simulink model "MultiLoop_mode1"  (Simulink 10.1)
settings: Solver=ode45  StartTime=0.0  StopTime=400  FixedStep=Ts_base  MinStep=1e-6  RelTol=1e-6
PreLoadFcn:
  | Mode_1_Init
StopFcn:
  | TEplot
values from neighbouring files (symbols this model uses):
  att_delay = 19.5    [convert_poison.m]
  att_idx = 1    [convert_poison.m]
  att_len = 3.0    (= 3)    [convert_poison.m]
  att_level = 22.9    [convert_poison.m]
  attack_gen_mode = 0    [convert_poison.m]
  n_poisons = 0    [convert_poison.m]
  poison_len = period * 5    (= 35.25)    [convert_poison.m]
  poisons = zeros( np, plen_ticks )    [convert_poison.m]
undefined symbols (not defined in the file or in its folder): r1_0, r4_0, Ts_base, Ts_save
libraries: TElib x17
settings Model: Creator=ricker  LastModifiedBy=mkrav  PacingRate=1.100000
settings DataIOCC: LoadInitialState=on  SaveFinalState=on  SaveFormat=Structure  SignalLoggingSaveFormat=ModelDataLogs  SaveOutput=off  SignalLogging=off  SaveTime=off  SignalLoggingName=sigsOut
settings OptimizationCC: InitFltsAndDblsToZero=on
settings DebuggingCC: SaveWithParameterizedLinksMsg=none  SignalResolutionControl=TryResolveAllWithWarning  MultiTaskDSMMsg=warning  MultiTaskCondExecSysMsg=none  FcnCallInpInsideContextMsg=warning
settings HardwareCC: TargetUnknown=on
settings GRTTargetCC: TargetFcnLib=ansi_tfl_tmw.mat
settings ConfigComp: CovSFcnEnable=off

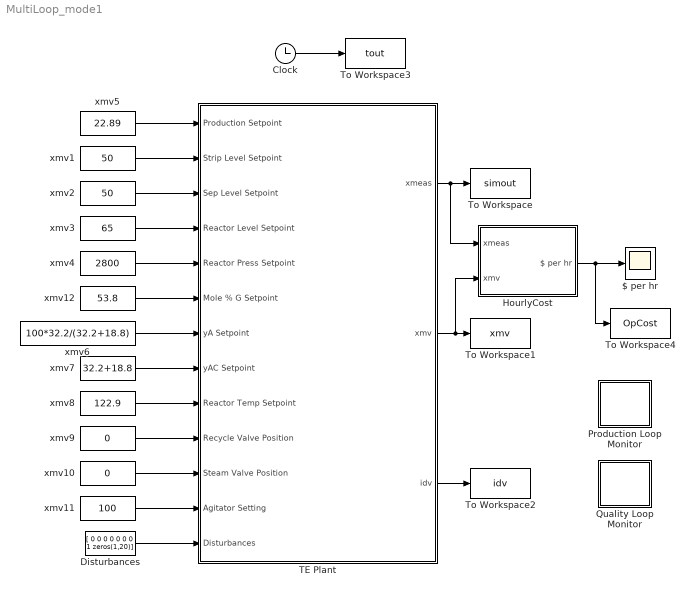
== system MultiLoop_mode1 ==
  $ per hr : Scope
  Clock : Clock
  Disturbances : Constant  Value=[ 0 0 0 0 0 0 0 1 zeros(1,20)]
  HourlyCost : Subsystem
  Production Loop Monitor : Subsystem
  Quality Loop Monitor : Subsystem
  TE Plant : Subsystem
  To Workspace : ToWorkspace  VariableName=simout  SampleTime=Ts_save
  To Workspace1 : ToWorkspace  VariableName=xmv  SampleTime=Ts_save
  To Workspace2 : ToWorkspace  VariableName=idv  SampleTime=Ts_save
  To Workspace3 : ToWorkspace  VariableName=tout  SampleTime=Ts_save
  To Workspace4 : ToWorkspace  VariableName=OpCost  SampleTime=Ts_save
  xmv1 : Constant  Value=50
  xmv10 : Constant  Value=0
  xmv11 : Constant  Value=100
  xmv12 : Constant  Value=53.8
  xmv2 : Constant  Value=50
  xmv3 : Constant  Value=65
  xmv4 : Constant  Value=2800
  xmv5 : Constant  Value=22.89
  xmv6 : Constant  Value=100*32.2/(32.2+18.8)
  xmv7 : Constant  Value=32.2+18.8
  xmv8 : Constant  Value=122.9
  xmv9 : Constant  Value=0
  wires:
  TE Plant/1(xmeas) -> To Workspace/1, HourlyCost/1(xmeas)
  xmv1/1 -> TE Plant/2(Strip Level Setpoint)
  xmv2/1 -> TE Plant/3(Sep Level Setpoint)
  xmv3/1 -> TE Plant/4(Reactor Level Setpoint)
  xmv4/1 -> TE Plant/5(Reactor Press Setpoint)
  xmv8/1 -> TE Plant/9(Reactor Temp Setpoint)
  xmv6/1 -> TE Plant/7(yA Setpoint)
  xmv7/1 -> TE Plant/8(yAC Setpoint)
  TE Plant/2(xmv) -> To Workspace1/1, HourlyCost/2(xmv)
  TE Plant/3(idv) -> To Workspace2/1
  Clock/1 -> To Workspace3/1
  HourlyCost/1($ per hr) -> $ per hr/1, To Workspace4/1
  xmv9/1 -> TE Plant/10(Recycle Valve Position)
  xmv10/1 -> TE Plant/11(Steam Valve Position)
  xmv11/1 -> TE Plant/12(Agitator Setting)
  Disturbances/1 -> TE Plant/13(Disturbances)
  xmv12/1 -> TE Plant/6(Mole % G Setpoint)
  xmv5/1 -> TE Plant/1(Production Setpoint)

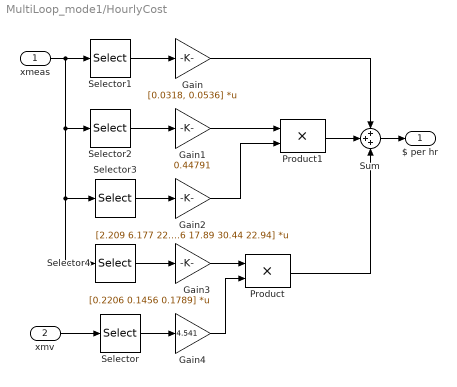
== system MultiLoop_mode1/HourlyCost ==
  xmeas : Inport  PortDimensions=41
  xmv : Inport  Port=2  PortDimensions=12
  Gain : Gain  Gain=[0.0318, 0.0536]  Multiplication=Matrix(K*u)  SaturateOnIntegerOverflow=on  OutDataTypeStr=Inherit: Same as input  ParamDataTypeStr=Inherit: Same as input
  Gain1 : Gain  Gain=0.44791  SaturateOnIntegerOverflow=on  OutDataTypeStr=Inherit: Same as input  ParamDataTypeStr=Inherit: Same as input
  Gain2 : Gain  Gain=[2.209 6.177 22.06 14.56 17.89 30.44 22.94]  Multiplication=Matrix(K*u)  SaturateOnIntegerOverflow=on  OutDataTypeStr=Inherit: Same as input  ParamDataTypeStr=Inherit: Same as input
  Gain3 : Gain  Gain=[0.2206 0.1456 0.1789]  Multiplication=Matrix(K*u)  SaturateOnIntegerOverflow=on  OutDataTypeStr=Inherit: Same as input  ParamDataTypeStr=Inherit: Same as input
  Gain4 : Gain  Gain=4.541  SaturateOnIntegerOverflow=on  OutDataTypeStr=Inherit: Same as input  ParamDataTypeStr=Inherit: Same as input
  Product : Product  SaturateOnIntegerOverflow=on  OutDataTypeStr=Inherit: Same as first input
  Product1 : Product  SaturateOnIntegerOverflow=on  OutDataTypeStr=Inherit: Same as first input
  Selector : Selector  InputPortWidth=12  IndexOptions=Index vector (dialog)  Indices=8  OutputSizes=1
  Selector1 : Selector  InputPortWidth=41  IndexOptions=Index vector (dialog)  Indices=[19 20]  OutputSizes=1
  Selector2 : Selector  InputPortWidth=41  IndexOptions=Index vector (dialog)  Indices=[10]  OutputSizes=1
  Selector3 : Selector  InputPortWidth=41  IndexOptions=Index vector (dialog)  Indices=[29, 31:36]  OutputSizes=1
  Selector4 : Selector  InputPortWidth=41  IndexOptions=Index vector (dialog)  Indices=[37:39]  OutputSizes=1
  Sum : Sum  Inputs=+++  SaturateOnIntegerOverflow=on
  $ per hr : Outport
  wires:
  xmv/1 -> Selector/1
  xmeas/1 -> Selector1/1, Selector2/1, Selector3/1, Selector4/1
  Selector1/1 -> Gain/1
  Selector2/1 -> Gain1/1
  Selector3/1 -> Gain2/1
  Selector4/1 -> Gain3/1
  Selector/1 -> Gain4/1
  Gain3/1 -> Product/1
  Gain4/1 -> Product/2
  Sum/1 -> $ per hr/1
  Product/1 -> Sum/3
  Gain/1 -> Sum/1
  Product1/1 -> Sum/2
  Gain1/1 -> Product1/1
  Gain2/1 -> Product1/2

== system MultiLoop_mode1/Production Loop Monitor ==
  Mux2 : Mux  Inputs=2
  Production : Scope
  wires:
  Mux2/1 -> Production/1
  [xmeas17] -> Mux2/2
  [Prodsp] -> Mux2/1

== system MultiLoop_mode1/Quality Loop Monitor ==
  Mux2 : Mux  Inputs=2
  Quality : Scope
  wires:
  [PctGsp] -> Mux2/1
  [xmeas40] -> Mux2/2
  Mux2/1 -> Quality/1

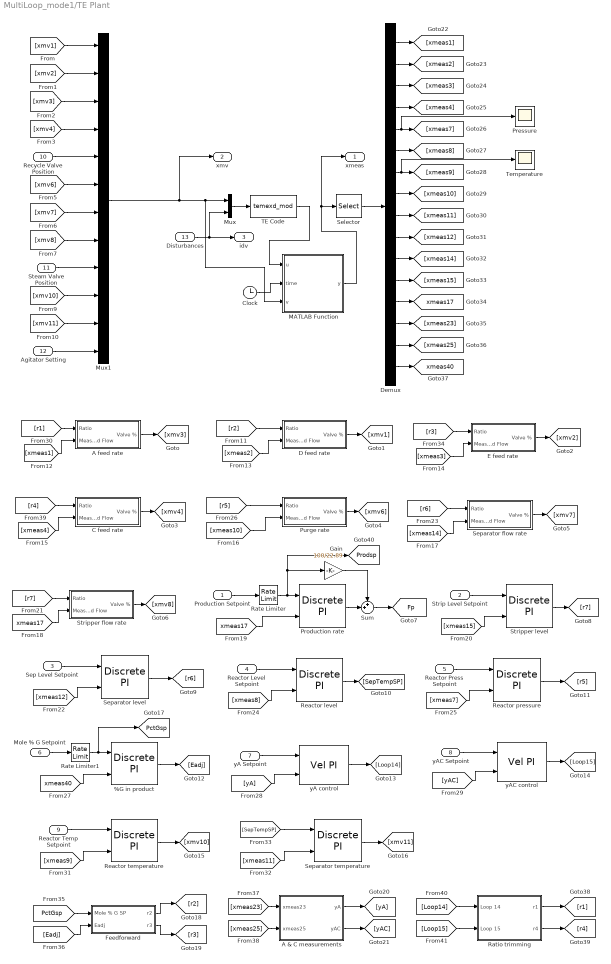
== system MultiLoop_mode1/TE Plant ==
  Production Setpoint : Inport
  Strip Level Setpoint : Inport  Port=2
  Sep Level Setpoint : Inport  Port=3
  Reactor Level Setpoint : Inport  Port=4
  Reactor Press Setpoint : Inport  Port=5
  Mole % G Setpoint : Inport  Port=6
  yA Setpoint : Inport  Port=7
  yAC Setpoint : Inport  Port=8
  Reactor Temp Setpoint : Inport  Port=9
  Recycle Valve Position : Inport  Port=10
  Steam Valve Position : Inport  Port=11
  Agitator Setting : Inport  Port=12
  Disturbances : Inport  Port=13
  %G in product : TElib/Discrete PI  Kc=-0.4  Ti=100/60  Ts=Ts_base  x0=Eadj_0  Hi=inf  Lo=-inf
  A & C measurements : Subsystem
  A feed rate : Subsystem
  C feed rate : Subsystem
  Clock : Clock
  D feed rate : Subsystem
  Demux : Demux  Outputs=16
      settings: DisplayOption=none
  E feed rate : Subsystem
  Feedforward : Subsystem
  Gain : Gain  Gain=100/22.89  SaturateOnIntegerOverflow=on  OutDataTypeStr=Inherit: Same as input  ParamDataTypeStr=Inherit: Same as input
  MATLAB Function : MATLAB Function  TreatAsAtomicUnit=on
  Mux : Mux  Inputs=2
  Mux1 : Mux  Inputs=12
  Pressure : Scope
  Production rate : TElib/Discrete PI  Kc=3.2  Ti=120/60  Ts=Ts_base  x0=0  Hi=30  Lo=-30
  Purge rate : Subsystem
  Rate Limiter : RateLimiter  RisingSlewLimit=0.3*22.95/24  FallingSlewLimit=-0.3*22.95/24
  Rate Limiter1 : RateLimiter  RisingSlewLimit=50/24  FallingSlewLimit=-50/24
  Ratio trimming : Subsystem
  Reactor level : TElib/Discrete PI  Kc=0.8  Ti=60/60  Ts=Ts_base  x0=SP17_0  Hi=120  Lo=0
  Reactor pressure : TElib/Discrete PI  Kc=-1e-4  Ti=20/60  Ts=Ts_base  x0=r5_0  Hi=100  Lo=0
  Reactor temperature : TElib/Discrete PI  Kc=-8  Ti=7.5/60  Ts=Ts_base  x0=xmv10_0  Hi=100  Lo=0
  Selector : Selector  InputPortWidth=41  IndexOptions=Index vector (dialog)  Indices=[1:4, 7:12, 14, 15, 17, 23, 25, 40]  OutputSizes=1
  Separator flow rate : Subsystem
  Separator level : TElib/Discrete PI  Kc=-1e-3  Ti=200/60  Ts=Ts_base  x0=r6_0  Hi=100  Lo=0
  Separator temperature : TElib/Discrete PI  Kc=-4  Ti=15/60  Ts=Ts_base  x0=xmv11_0  Hi=100  Lo=0
  Stripper flow rate : Subsystem
  Stripper level : TElib/Discrete PI  Kc=-2e-4  Ti=200/60  Ts=Ts_base  x0=r7_0  Hi=100  Lo=0
  Sum : Sum  Inputs=++|  SaturateOnIntegerOverflow=on
  TE Code : S-Function  FunctionName=temexd_mod  SFunctionDeploymentMode=off  EnableBusSupport=off
  Temperature : Scope
  yA control : TElib/Discrete PI/Vel PI  Kc=2e-4  Ti=1  Ts=0.1
  yAC control : TElib/Discrete PI/Vel PI  Kc=3e-4  Ti=2  Ts=0.1
  xmeas : Outport
  xmv : Outport  Port=2
  idv : Outport  Port=3
  tag scope: Fp=global, PctGsp=global, Prodsp=global, xmeas17=global, xmeas40=global
  wires:
  Mux/1 -> TE Code/1
  Disturbances/1 -> Mux/2, idv/1
  TE Code/1 -> MATLAB Function/1(u)
  [xmv1] -> Mux1/1
  [xmv2] -> Mux1/2
  [xmv3] -> Mux1/3
  [xmv4] -> Mux1/4
  Recycle Valve Position/1 -> Mux1/5
  [xmv6] -> Mux1/6
  [xmv7] -> Mux1/7
  [xmv8] -> Mux1/8
  Steam Valve Position/1 -> Mux1/9
  [xmv10] -> Mux1/10
  [xmv11] -> Mux1/11
  Agitator Setting/1 -> Mux1/12
  A feed rate/1(Valve %) -> [xmv3]
  [xmeas1] -> A feed rate/2(Measured Flow)
  D feed rate/1(Valve %) -> [xmv1]
  [xmeas2] -> D feed rate/2(Measured Flow)
  E feed rate/1(Valve %) -> [xmv2]
  [xmeas3] -> E feed rate/2(Measured Flow)
  C feed rate/1(Valve %) -> [xmv4]
  [xmeas4] -> C feed rate/2(Measured Flow)
  Purge rate/1(Valve %) -> [xmv6]
  [xmeas10] -> Purge rate/2(Measured Flow)
  Separator flow rate/1(Valve %) -> [xmv7]
  [xmeas14] -> Separator flow rate/2(Measured Flow)
  Stripper flow rate/1(Valve %) -> [xmv8]
  [xmeas17] -> Stripper flow rate/2(Measured Flow)
  [xmeas17] -> Production rate/2
  [xmeas15] -> Stripper level/2
  Strip Level Setpoint/1 -> Stripper level/1
  Stripper level/1 -> [r7]
  [r7] -> Stripper flow rate/1(Ratio)
  [xmeas12] -> Separator level/2
  Sep Level Setpoint/1 -> Separator level/1
  Separator level/1 -> [r6]
  [r6] -> Separator flow rate/1(Ratio)
  [xmeas8] -> Reactor level/2
  Reactor Level Setpoint/1 -> Reactor level/1
  Reactor level/1 -> [SepTempSP]
  [xmeas7] -> Reactor pressure/2
  Reactor Press Setpoint/1 -> Reactor pressure/1
  Reactor pressure/1 -> [r5]
  [r5] -> Purge rate/1(Ratio)
  [xmeas40] -> %G in product/2
  %G in product/1 -> [Eadj]
  [yA] -> yA control/2
  yA Setpoint/1 -> yA control/1
  yA control/1 -> [Loop14]
  [yAC] -> yAC control/2
  yAC Setpoint/1 -> yAC control/1
  yAC control/1 -> [Loop15]
  [r1] -> A feed rate/1(Ratio)
  [xmeas9] -> Reactor temperature/2
  Reactor Temp Setpoint/1 -> Reactor temperature/1
  Reactor temperature/1 -> [xmv10]
  [xmeas11] -> Separator temperature/2
  [SepTempSP] -> Separator temperature/1
  Separator temperature/1 -> [xmv11]
  [r2] -> D feed rate/1(Ratio)
  [r3] -> E feed rate/1(Ratio)
  [PctGsp] -> Feedforward/1(Mole % G SP)
  [Eadj] -> Feedforward/2(Eadj)
  Feedforward/1(r2) -> [r2]
  Feedforward/2(r3) -> [r3]
  [xmeas23] -> A & C measurements/1(xmeas23)
  [xmeas25] -> A & C measurements/2(xmeas25)
  A & C measurements/1(yA) -> [yA]
  A & C measurements/2(yAC) -> [yAC]
  Mux1/1 -> MATLAB Function/3(v), Mux/1, xmv/1
  Selector/1 -> Demux/1
  Demux/1 -> [xmeas1]
  Demux/2 -> [xmeas2]
  Demux/3 -> [xmeas3]
  Demux/4 -> [xmeas4]
  Demux/5 -> [xmeas7], Pressure/1
  Demux/6 -> [xmeas8]
  Demux/7 -> [xmeas9], Temperature/1
  Demux/8 -> [xmeas10]
  Demux/9 -> [xmeas11]
  Demux/10 -> [xmeas12]
  Demux/11 -> [xmeas14]
  Demux/12 -> [xmeas15]
  Demux/13 -> [xmeas17]
  Demux/14 -> [xmeas23]
  Demux/15 -> [xmeas25]
  Demux/16 -> [xmeas40]
  [r4] -> C feed rate/1(Ratio)
  [Loop14] -> Ratio trimming/1(Loop 14)
  [Loop15] -> Ratio trimming/2(Loop 15)
  Ratio trimming/1(r1) -> [r1]
  Ratio trimming/2(r4) -> [r4]
  Production Setpoint/1 -> Rate Limiter/1
  Rate Limiter/1 -> Production rate/1, [Prodsp], Gain/1
  Mole % G Setpoint/1 -> Rate Limiter1/1
  Rate Limiter1/1 -> %G in product/1, [PctGsp]
  Production rate/1 -> Sum/2
  Sum/1 -> [Fp]
  Gain/1 -> Sum/1
  MATLAB Function/1(y) -> xmeas/1, Selector/1
  Clock/1 -> MATLAB Function/2(time)

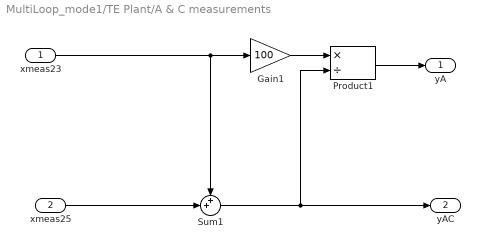
== system MultiLoop_mode1/TE Plant/A & C measurements ==
  xmeas23 : Inport
  xmeas25 : Inport  Port=2
  Gain1 : Gain  Gain=100  SaturateOnIntegerOverflow=on  OutDataTypeStr=Inherit: Same as input  ParamDataTypeStr=Inherit: Same as input
  Product1 : Product  Inputs=*/  SaturateOnIntegerOverflow=on  OutDataTypeStr=Inherit: Same as first input
  Sum1 : Sum  Inputs=++|  SaturateOnIntegerOverflow=on
  yA : Outport
  yAC : Outport  Port=2
  wires:
  Sum1/1 -> yAC/1, Product1/2
  xmeas23/1 -> Sum1/1, Gain1/1
  xmeas25/1 -> Sum1/2
  Gain1/1 -> Product1/1
  Product1/1 -> yA/1

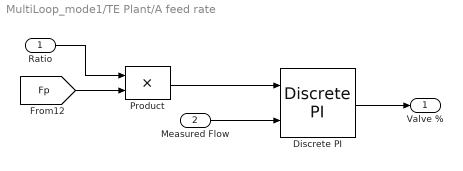
== system MultiLoop_mode1/TE Plant/A feed rate ==
  Ratio : Inport
  Measured Flow : Inport  Port=2
  Discrete PI : TElib/Discrete PI  Kc=0.01  Ti=0.001/60  Ts=Ts_base  x0=xmv3_0  Hi=100  Lo=0
  Product : Product  SaturateOnIntegerOverflow=on  OutDataTypeStr=Inherit: Same as first input
  Valve % : Outport
  wires:
  Discrete PI/1 -> Valve %/1
  Ratio/1 -> Product/1
  [Fp] -> Product/2
  Measured Flow/1 -> Discrete PI/2
  Product/1 -> Discrete PI/1

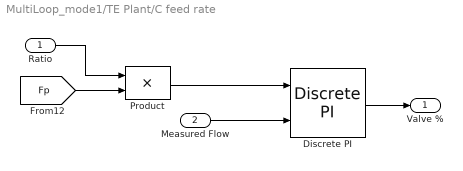
== system MultiLoop_mode1/TE Plant/C feed rate ==
  Ratio : Inport
  Measured Flow : Inport  Port=2
  Discrete PI : TElib/Discrete PI  Kc=0.003  Ti=0.001/60  Ts=Ts_base  x0=xmv4_0  Hi=100  Lo=0
  Product : Product  SaturateOnIntegerOverflow=on  OutDataTypeStr=Inherit: Same as first input
  Valve % : Outport
  wires:
  Product/1 -> Discrete PI/1
  Measured Flow/1 -> Discrete PI/2
  [Fp] -> Product/2
  Ratio/1 -> Product/1
  Discrete PI/1 -> Valve %/1

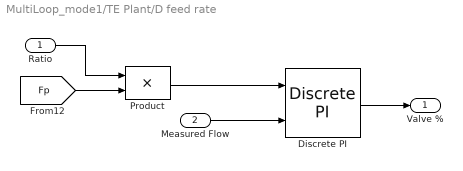
== system MultiLoop_mode1/TE Plant/D feed rate ==
  Ratio : Inport
  Measured Flow : Inport  Port=2
  Discrete PI : TElib/Discrete PI  Kc=1.6e-6  Ti=0.001/60  Ts=Ts_base  x0=xmv1_0  Hi=100  Lo=0
  Product : Product  SaturateOnIntegerOverflow=on  OutDataTypeStr=Inherit: Same as first input
  Valve % : Outport
  wires:
  Product/1 -> Discrete PI/1
  Measured Flow/1 -> Discrete PI/2
  [Fp] -> Product/2
  Ratio/1 -> Product/1
  Discrete PI/1 -> Valve %/1

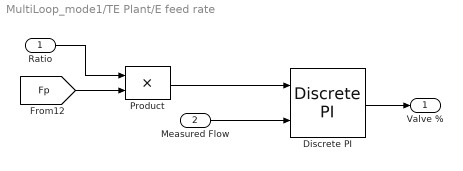
== system MultiLoop_mode1/TE Plant/E feed rate ==
  Ratio : Inport
  Measured Flow : Inport  Port=2
  Discrete PI : TElib/Discrete PI  Kc=1.8e-6  Ti=0.001/60  Ts=Ts_base  x0=xmv2_0  Hi=100  Lo=0
  Product : Product  SaturateOnIntegerOverflow=on  OutDataTypeStr=Inherit: Same as first input
  Valve % : Outport
  wires:
  Product/1 -> Discrete PI/1
  Measured Flow/1 -> Discrete PI/2
  [Fp] -> Product/2
  Ratio/1 -> Product/1
  Discrete PI/1 -> Valve %/1

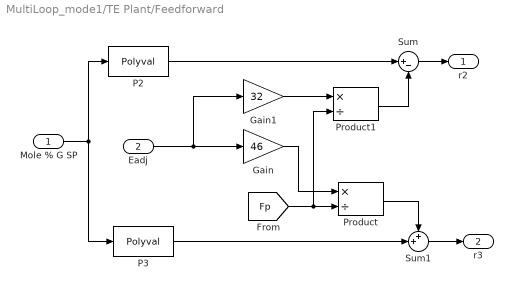
== system MultiLoop_mode1/TE Plant/Feedforward ==
  Mole % G SP : Inport
  Eadj : Inport  Port=2
  Gain : Gain  Gain=46  SaturateOnIntegerOverflow=on  OutDataTypeStr=Inherit: Same as input  ParamDataTypeStr=Inherit: Same as input
  Gain1 : Gain  Gain=32  SaturateOnIntegerOverflow=on  OutDataTypeStr=Inherit: Same as input  ParamDataTypeStr=Inherit: Same as input
  P2 : Polyval  Coefs="[1.5192e-003  5.9446e-001  2.7690e-001]"
  P3 : Polyval  Coefs="[-1.1377e-003 -8.0893e-001  9.1060e+001]"
  Product : Product  Inputs=*/  SaturateOnIntegerOverflow=on  OutDataTypeStr=Inherit: Same as first input
  Product1 : Product  Inputs=*/  SaturateOnIntegerOverflow=on  OutDataTypeStr=Inherit: Same as first input
  Sum : Sum  Inputs=|+-  SaturateOnIntegerOverflow=on
  Sum1 : Sum  Inputs=++|  SaturateOnIntegerOverflow=on
  r2 : Outport
  r3 : Outport  Port=2
  wires:
  Mole % G SP/1 -> P2/1, P3/1
  Sum/1 -> r2/1
  P2/1 -> Sum/1
  Sum1/1 -> r3/1
  P3/1 -> Sum1/2
  Product/1 -> Sum1/1
  [Fp] -> Product/2, Product1/2
  Gain/1 -> Product/1
  Eadj/1 -> Gain/1, Gain1/1
  Product1/1 -> Sum/2
  Gain1/1 -> Product1/1

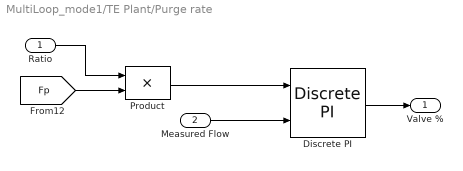
== system MultiLoop_mode1/TE Plant/Purge rate ==
  Ratio : Inport
  Measured Flow : Inport  Port=2
  Discrete PI : TElib/Discrete PI  Kc=0.01  Ti=0.001/60  Ts=Ts_base  x0=xmv6_0  Hi=100  Lo=0
  Product : Product  SaturateOnIntegerOverflow=on  OutDataTypeStr=Inherit: Same as first input
  Valve % : Outport
  wires:
  Discrete PI/1 -> Valve %/1
  Ratio/1 -> Product/1
  [Fp] -> Product/2
  Measured Flow/1 -> Discrete PI/2
  Product/1 -> Discrete PI/1

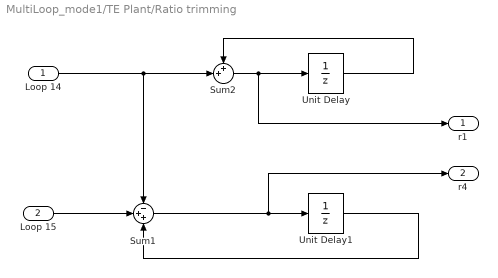
== system MultiLoop_mode1/TE Plant/Ratio trimming ==
  Loop 14 : Inport
  Loop 15 : Inport  Port=2
  Sum1 : Sum  Inputs=-++  SaturateOnIntegerOverflow=on
  Sum2 : Sum  Inputs=++|  SaturateOnIntegerOverflow=on
  Unit Delay : UnitDelay  InitialCondition=r1_0  SampleTime=0.1  HasFrameUpgradeWarning=on
  Unit Delay1 : UnitDelay  InitialCondition=r4_0  SampleTime=0.1  HasFrameUpgradeWarning=on
  r1 : Outport
  r4 : Outport  Port=2
  wires:
  Loop 15/1 -> Sum1/2
  Unit Delay/1 -> Sum2/1
  Unit Delay1/1 -> Sum1/3
  Sum2/1 -> Unit Delay/1, r1/1
  Loop 14/1 -> Sum2/2, Sum1/1
  Sum1/1 -> Unit Delay1/1, r4/1

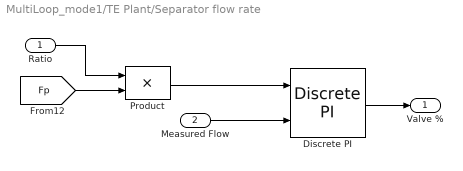
== system MultiLoop_mode1/TE Plant/Separator flow rate ==
  Ratio : Inport
  Measured Flow : Inport  Port=2
  Discrete PI : TElib/Discrete PI  Kc=4e-4  Ti=0.001/60  Ts=Ts_base  x0=xmv7_0  Hi=100  Lo=0
  Product : Product  SaturateOnIntegerOverflow=on  OutDataTypeStr=Inherit: Same as first input
  Valve % : Outport
  wires:
  Product/1 -> Discrete PI/1
  Measured Flow/1 -> Discrete PI/2
  [Fp] -> Product/2
  Ratio/1 -> Product/1
  Discrete PI/1 -> Valve %/1

== system MultiLoop_mode1/TE Plant/Stripper flow rate ==
  Ratio : Inport
  Measured Flow : Inport  Port=2
  Discrete PI : TElib/Discrete PI  Kc=4e-4  Ti=0.001/60  Ts=Ts_base  x0=xmv8_0  Hi=100  Lo=0
  Product : Product  SaturateOnIntegerOverflow=on  OutDataTypeStr=Inherit: Same as first input
  Valve % : Outport
  wires:
  Discrete PI/1 -> Valve %/1
  Ratio/1 -> Product/1
  [Fp] -> Product/2
  Measured Flow/1 -> Discrete PI/2
  Product/1 -> Discrete PI/1

== matlab function TE Plant/MATLAB Function ==
  settings: updateMethod=DISCRETE
  data: u input double; y output double; time input double; v input double; poisons parameter double; att_delay parameter double; att_level parameter double; attack_gen_mode parameter double; att_idx parameter double; n_poisons parameter double; poison_len parameter double; att_len parameter double
% data arrives from the file syncronized with the simulation clock like
% this:
% load("../te_attack_3_poison0.mat")
% s = size(p_xmeas_13)
% times = linspace(0,20,s(1,2))
% ts = timeseries(p_xmeas_13, times)
% save te_attack3_poison.mat -v7.3 ts

% To add more parameters from the MATLAB workspace use Modeling->Model
% Explorer
function y = fcn(u, time, v, poisons, att_delay, att_level, attack_gen_mode, att_idx, n_poisons, poison_len, att_len)
    coder.extrinsic('py.array.array')    
    coder.extrinsic('py.LR_pred.load_model')    
    coder.extrinsic('py.LR_pred.predict')
    % determined analytically, would be good to confirm based on the 
    % simulation parameters. TODO - get from the workspace
    period = 7.05;
    plen_ticks = poison_len * 10000;
    
    tick_idx = time * 10000; % while we get the call every 0.0005, we save the poisons at resolution of 0.0001
    poison_idx = fix(tick_idx / plen_ticks) + 1;
    tick_idx = rem(tick_idx, plen_ticks) + 1;

    % Reactor pressure shutdown
    % the controller is trying to keep the value at its setpoint
    % the setpoint, r1 is set in Mode_1_Init.m r1_0=0.251
    % When set to 2 and above the valve will close and the reactor will shut down
    % in 6 hours, exactly as in the IDV 6
    % Nice: if (time > 1) && (time < 9) causes the system to get into
    % unstable state and shut down few hours later
    % Attack 1
%     if (time > 1) && (time < 9) 
%         % this will make it easier for me to find the real value
%         % TODO - output the  real values too
%         u(1) = u(1) + 3; 
%     end
    %p_mat = load_poison(time);
   % fprintf("Called at time %f\n", time); 
   persistent att_end;
   persistent att_demo_end;
   persistent in_poison;
   persistent in_attack;
   persistent curr_poison;
   persistent curr_poison_tick;
   persistent prev_pred;
   if isempty(curr_poison)
       % The first time initialization
       curr_poison = 1;
       curr_poison_tick = 0;
       prev_pred = 1.0;
       py.LR_pred.load_model(sprintf("_te_attack_%d", int8(att_idx)));
   end
   % I still do not understand why the attack's effect is so widely
   % different and what is it dependent on
   % I noticed that the tefunc is called 15 time more frequent than this
   % function
   % Steps of attack timing tuning:
   % 1. Decrease the att_len in the attack generation mode until the
   % shutdown disappears
   % 2. Find the lowest att_margin that still causes the shutdown from the 
   % attack in the non-generation mode. Do it with the correct poison, 
   % otherwise you'll have to adjust it
   % att_len = 0;
   att_margin = 0;
   %att_level = 0;
   if att_idx == 1
        %att_len = 5;%2.54;%7.19;% 5.84; % Attack 1
        att_margin = 0.05;%4.65;%0.02; % Attack 1 ? 
   elseif att_idx == 2
        att_len = 2.88; % Attack 2
        att_margin = 0.053; % Attack 2
   elseif att_idx == 21
        att_len = 2.6; % Holding attack 2
        % check if needs to be different from 2
        att_margin = 0.01; 
   elseif att_idx == 31
        att_len = 1.9;%1.9295;%1.87;%1.9295; %3.17; %1.9295; %1.98; % Holding attacks 3
        % We should change u(12) instead of u(15) - check next 
        att_margin = 0.05;%0.03;%0.02;%0.05; %Seems too large...
   elseif att_idx == 3
        att_len = 2.02; % Attack 3
        att_margin = 0.02; % Attack 3
   end
   
   % att_margin: should be as small as possible while:
   % 1. causing the shutdown FROM THE ATTACK with attack_gen_mode = 0
   % 2. not causing the shutdown with attack_gen_mode = 1
   % Setting
   rel_att_magn = att_level;%7;
   rel_att_start = period;
   rel_att_end = rel_att_start + att_len - att_margin;
   if attack_gen_mode == 0
       poison_delay = att_delay;
       poison_prob_thresh = 0.4;
       if att_idx == 31
           poison_delay = 19.5;
       elseif att_idx == 1
           poison_prob_thresh = 0.2;
           poison_delay = 6; 
       elseif att_idx == 2
           poison_delay = 0;
       elseif att_idx == 3
           poison_delay = 0;
           % poison_prob_thresh = 0.2;
           % NOTE that the presented number of alerts was measured without
           % any contraint on the poison. When using 0.4 it comes out a bit
           % smaller
       end
       
%        fprintf("time %f poison_idx %f tick_idx %f\n", time, poison_idx, tick_idx);
       att_start_tick = (rel_att_start + poison_delay) * 10000;

       % if I haven't completed the current poison yet
       apply_poison = false;
       if curr_poison <= poison_idx && time < (n_poisons * poison_len) && ...
             rem(time, poison_len) > rel_att_start + poison_delay %% + att_delayTEMP TEMP
           %- for PP training - allows me to allpy the poison after the
           % specified delay to get a complete coverage
           poison_level = poisons(poison_idx, att_start_tick);
           if att_idx == 1
               % TODO - check the precise ticks after adding the predictor
               poison_level = poisons(poison_idx, att_start_tick) - poisons(poison_idx, att_start_tick - 100); 
           elseif att_idx == 2
               % TODO - check the precise ticks 
               % using +130 was found empirically, as the largest
               % difference
               % and is wrong to use! the largest difference is due to the
               % interpolation and is larger than intended!
               poison_level = poisons(poison_idx, att_start_tick + 130) - poisons(poison_idx, att_start_tick); 
           elseif att_idx == 3
               % due to rounding error the attack starts 2 timepoints
               % earlier
               att_start_tick = att_start_tick - 200;
               poison_level = poisons(poison_idx, att_start_tick) - poisons(poison_idx, att_start_tick + 100); 
           end
           % if we are not in the middle of applying the poison 
           if isempty(in_poison)
               % check if applying the poison now is safe
                pred = prev_pred;
                if att_idx == 1
                    pred = double(py.LR_pred.predict([poison_level u(1) u(7) u(8) v(3) att_len - att_margin]));
                else
                    pred = double(py.LR_pred.predict([poison_level u(12) u(14) v(7) u(15) u(17) v(8) att_len - att_margin]));
                end
                if pred < poison_prob_thresh && prev_pred < poison_prob_thresh
                    in_poison = 1;
                    curr_poison_tick = 1;
                    apply_poison = true;
                    fprintf("poison_idx %f tick_idx %f\n",poison_idx, tick_idx);
                    if att_idx == 1
                        fprintf("Applying poison with A Feed Rate u(1) %f, Reactor Pressure u(7) %f, Reactor Level u8 %f, xmv3 %f at time %f\n", u(1), u(7), u(8), v(3), time);
                    else
                        fprintf("Applying poison with Sep level u(12) %f, Sep flow u(14) %f, xmv7 %f, Strip level u(15) %f, strip flow u(17) %f xmv8 %f at time %f\n", u(12), u(14), v(7), u(15), u(17), v(8), time);
                    end
                end
                prev_pred = pred;
           % if we are not in the middle of applying the poison 
           elseif in_poison == 0
               % check if applying the poison now is safe
                pred = prev_pred;
                if att_idx == 1
                    pred = double(py.LR_pred.predict([poison_level u(1) u(7) u(8) v(3) att_len - att_margin]));
                else
                    pred = double(py.LR_pred.predict([poison_level u(12) u(14) v(7) u(15) u(17) v(8) att_len - att_margin]));
                end
                if pred < poison_prob_thresh && prev_pred < poison_prob_thresh
                    in_poison = 1;
                    curr_poison_tick = 1;
                    apply_poison = true;
                    fprintf("poison_idx %f tick_idx %f\n",poison_idx, tick_idx);
                    if att_idx == 1
                        fprintf("Applying poison with A Feed Rate u(1) %f, Reactor Pressure u(7) %f, Reactor Level u8 %f, xmv3 %f at time %f\n", u(1), u(7), u(8), v(3), time);
                    else
                        fprintf("Applying poison with Sep level u(12) %f, Sep flow u(14) %f, xmv7 %f, Strip level u(15) %f, strip flow u(17) %f xmv8 %f at time %f\n", u(12), u(14), v(7), u(15), u(17), v(8), time);
                    end
                end
                prev_pred = pred;
           elseif in_poison == 1
               %fprintf("curr_poison_tick %f time %f\n", curr_poison_tick, time);
               % should we stop?
               if curr_poison_tick > (att_len - att_margin) * 10000
                   in_poison = 0;
                   curr_poison = curr_poison + 1;
                    if att_idx == 1
                        fprintf("Stop applying poison with A Feed Rate u(1) %f, Reactor Pressure u(7) %f, Reactor Level u8 %f, xmv3 %f at time %f\n", u(1), u(7), u(8), v(3), time);
                    else
                        fprintf("Stop applying poison with Sep level u(12) %f, Sep flow u(14) %f, xmv7 %f, Strip level u(15) %f, strip flow u(17) %f xmv8 %f at time %f\n", u(12), u(14), v(7), u(15), u(17), v(8), time);
                    end
               else
                   apply_poison = true;
                   curr_poison_tick = curr_poison_tick + 5; % saved at higher resolution
               end
               prev_pred = 1.0;
           end
           if apply_poison
               if att_idx == 1
                    u(1) = poisons(poison_idx, att_start_tick + curr_poison_tick - 1);
               else
                    u(14) = poisons(poison_idx, att_start_tick + curr_poison_tick - 1);
               end
           end
       end
       
        % IMPORTANT:
        % 1. Apply the attack ONLY when we carry out the actual change, not
        % more, otherwise system goes astray
        % 2. Make sure to apply it for no longer that the original attack

        %att_len = att_len - att_margin; %%TEMP TEMP - for PP training only
        att_start = (n_poisons * poison_len) + rel_att_start + att_delay;
        %     % att_start = period * 6 + 1;
        % %    if (time > att_start) && (time < att_start + 3) - Attack 3
        if (time > att_start)
           start_attack = 0; 
           if att_idx == 1 && isempty(att_end) 
                pred = prev_pred;
                pred = double(py.LR_pred.predict([att_level u(1) u(7) u(8) v(3) att_len]));
                if pred > 0.9%0.84 %&& prev_pred > 0.8 
                    start_attack = 1;
                end
           elseif att_idx == 2 && isempty(att_end) %&& u(14) > 25.5 && u(15) > 45.9 && u(15) < 45.98 % Attack 2
                pred = prev_pred;
                pred = double(py.LR_pred.predict([att_level u(12) u(14) v(7) u(15) u(17) v(8) att_len ]));
                if pred > 0.8 && prev_pred > 0.8 %0.93% 0.86 
                    start_attack = 1;
                end
           % 31 
           % Attack generation: Attacking with u(12) 53.490276 u(14) 25.570728 u(15) 45.971546 at time 7.050500
           % Stopping Attack generation: with u(12) 2.821349 u(14) 27.432461 u(15) 108.632118 at time 8.990500
           elseif att_idx == 3 && isempty(att_end) %&& u(14) < 25.6 && u(15) > 45.9 && u(15) < 45.98 % Attack 3
                pred = prev_pred;
                pred = double(py.LR_pred.predict([att_level u(12) u(14) v(7) u(15) u(17) v(8) att_len ]));
                if pred > 0.8 && prev_pred > 0.8 %0.93% 0.86 
                    start_attack = 1;
                end
%            elseif att_idx == 31 && isempty(att_end) && u(12) > 53.49 && u(12) < 53.50 && u(14) > 25.57 && u(14) < 25.59 && u(15) > 45.4% Attack 31
           elseif att_idx == 31 && isempty(att_end)% Attack 31
                pred = prev_pred;
                pred = double(py.LR_pred.predict([att_level u(12) u(14) v(7) u(15) u(17) v(8) att_len ]));
                if pred > 0.9 && prev_pred > 0.9 %0.93% 0.86
                    start_attack = 1;
                end
                prev_pred = pred;
           end
           if start_attack == 1
                att_start = time - att_margin;
                att_end = time + att_len; 
                in_attack = 1;
                if att_idx == 1
                    fprintf("Attacking with A Feed Rate u(1) %f, Reactor Pressure u(7) %f, Reactor Level u8 %f, xmv3 %f at time %f\n", u(1), u(7), u(8), v(3), time);
                else
                    fprintf("Attacking with Sep level u(12) %f, Sep flow u(14) %f, xmv7 %f, Strip level u(15) %f, strip flow u(17) %f xmv8 %f at time %f\n", u(12), u(14), v(7), u(15), u(17), v(8), time);
                end
           end
        end
        if (time > att_start) && ~isempty(att_end) && (time < att_end)  
            if att_idx == 1
                % Attack 1
                u(1) = u(1) + rel_att_magn;
            elseif att_idx == 2
                % Attack 2
                u(14) = u(14) + rel_att_magn;
            elseif att_idx == 3
                % Attack 3
                u(14) = u(14) - rel_att_magn;
            elseif att_idx == 31
                % Holding Attack 3
                % Pulling down Sep flow (u14) we cause the Separator valve
                % (xmv7) to open. This causes: Sep level (u12) going down
                % and Stripper level (u15) to go up. Sep level causes the
                % sep valve (xmv7) to close thus driving the stripper level
                % and flow. In addition, strip flow also influences the sep
                % valve to keep the production rate at the desired level
                % u(14) = att_level - 0.25;
                u(14) = att_level;
            end
        elseif ~isempty(att_end) && time >= att_end && ~isempty(in_attack) && in_attack == 1
            in_attack = 0;
            if att_idx == 1
                fprintf("Stop attacking poison with A Feed Rate u(1) %f, Reactor Pressure u(7) %f, Reactor Level u8 %f, xmv3 %f at time %f\n", u(1), u(7), u(8), v(3), time);
            else
                fprintf("Stop attacking poison with Sep level u(12) %f, Sep flow u(14) %f, xmv7 %f, Strip level u(15) %f, strip flow u(17) %f xmv8 %f at time %f\n", u(12), u(14), v(7), u(15), u(17), v(8), time);
            end
        end
   elseif attack_gen_mode == 1 % ATTACK GENERATION
       att_demo_start = rel_att_start + att_delay + n_poisons * poison_len;
       % After getting a working attack, subtract the margin and get the
       % attack to be use for poison generation (there we want "almost the
       % attack" so it is long and of the correct length)
       % att_margin = 0;
       if (time > att_demo_start)
           if isempty(att_demo_end)
                pred = prev_pred;
                if att_idx == 1
                    pred = double(py.LR_pred.predict([att_level u(1) u(7) u(8) v(3) att_len - att_margin]));
                else
                    pred = double(py.LR_pred.predict([att_level u(12) u(14) v(7) u(15) u(17) v(8) att_len - att_margin]));
                end
%                if pred > 0.86
%                 fprintf("Predicted %f\n", pred);
                    att_demo_start = time;
                    % first create an attack, then reduce it by att_margin so that
                    % that it does not happen and record
                    att_demo_end = time + att_len - att_margin;
                    in_poison = 1;
                    if att_idx == 1
                        fprintf("Attack generation with A Feed Rate u(1) %f, Reactor Pressure u(7) %f, Reactor Level u8 %f, xmv3 %f at time %f att_level %f\n", u(1), u(7), u(8), v(3), time, att_level);
                    else
                        fprintf("Attack generation with Sep level u(12) %f, Sep flow u(14) %f, xmv7 %f, Strip level u(15) %f, strip flow u(17) %f xmv8 %f at time %f att_level %f\n", u(12), u(14), v(7), u(15), u(17), v(8), time, att_level);
                    end
%               end
           end
       end
       if (time >= att_demo_start)  && ~isempty(att_demo_end) && (time < att_demo_end) 
            if att_idx == 1
                % Attack 2
                u(1) = u(1) + rel_att_magn;
            elseif att_idx == 2
                % Attack 2
                u(14) = u(14) + rel_att_magn;
            elseif att_idx == 21
                % Holding attack 2
                u(14) = 25.5 + 3.13;
            elseif att_idx == 31
                % Holding attack 3
                % Creating an attack that will work with and without poison
                % is very tricky.
                % Especially with holding attacks.
                % 1. Search for the right magnitude to cause the
                % shutdown.
                % 2. Check the length of the effective attack until the
                % system shuts down and set the att_len. Perform this with
                % att_margin = 0.
                % 3. Start increasing att_margin until the attack
                % disappears.
                u(14) = att_level;
            elseif att_idx == 3
                % Attack 3
                u(14) = u(14) - rel_att_magn;
            end
        elseif ~isempty(in_poison)
            if in_poison == 1
                if att_idx == 1
                    fprintf("Stop attack generation with A Feed Rate u(1) %f, Reactor Pressure u(7) %f, Reactor Level u8 %f, xmv3 %f at time %f\n", u(1), u(7), u(8), v(3), time);
                else
                    fprintf("Stop attack generation with Sep level u(12) %f, Sep flow u(14) %f, xmv7 %f, Strip level u(15) %f, strip flow u(17) %f xmv8 %f at time %f\n", u(12), u(14), v(7), u(15), u(17), v(8), time);
                end
                in_poison = 0;
            end
        end
   elseif attack_gen_mode == 2 % TRAIN_FOR_ATTACK GENERATION
       %simply apply partial attack every poison_len
       att_demo_start = rel_att_start + att_delay + n_poisons * poison_len;
%        apply_attack = (time >= att_demo_start) && rem(time, poison_len) > rel_att_start && rem(time, poison_len) < rel_att_start + att_len; 
       apply_attack = (time >= att_demo_start) && ...
           rem(time, poison_len) > rel_att_start ...
           && rem(time, poison_len) < rel_att_start + att_len - att_margin; 
       if apply_attack 
            if att_idx == 1
%                 u(1) = u(1) + rel_att_magn%/3;
                u(1) = u(1) + rel_att_magn;
            elseif att_idx == 2
                u(14) = u(14) + rel_att_magn/2;
            elseif att_idx == 21
                u(14) = 25.5 + 3.13/2;
            elseif att_idx == 31
                u(14) = att_level/2;
            elseif att_idx == 3
                % Attack 3
                u(14) = u(14) - rel_att_magn/2;
            end
        end
   end

    % Separator high level shutdown (normally 24 - 26.5, setpoint 0.2516)
    % Planned, but with XMEAS(14) = 50 really exited on Low Stripper Liquid Level!!  Shutting down.
    % Using values > 28 still causes it to quit on Low Stripper first
    % Using 27 causes High Stripper Liquid Level!!  Shutting down instead
    % u(14) = 27; I can't find a way to make it shut down after the attack
    % has completed.
    
    % Stripper low level shutdown (setpoint equivalent to 23) 
    % u(17) = 0;

    % Stripper high level shutdown (setpoint equivalent to 23) 
    % Setting it above 23 causes high level shutdown (high flow causes
    % the valve to close)
    % Keeping it at 23 produces nice effects, eventually exits with
    %  Low Stripper Liquid Level!!  Shutting down.
    % u(17) = 23.0;

y = u;
